simulink model "trajectory_traking"  (R2022b)
settings: Solver=ode4  StartTime=0.0  StopTime=T-T/duration  FixedStep=T/duration  RelTol=1e-3
values from neighbouring files (symbols this model uses):
  A = [ ... (first row only)    [path_generation.m]    (also in pid_test.m; trajectory.m)
  B = [ ... (first row only)    [path_generation.m]    (also in pid_test.m; trajectory.m)
  C = eye(4)    [path_generation.m]    (also in pid_test.m; trajectory.m)
  D = zeros(4,2)    [path_generation.m]    (also in pid_test.m; trajectory.m)
  Kd = 10*eye(4,2)    [drone.m]    (also in path_generation.m = K(:,3:4); trajectory.m = K(:,3:4))
  Kp = 20*eye(4,2)    [drone.m]    (also in path_generation.m = K(:,1:2); trajectory.m = K(:,1:2))
  x0 = [ ... (first row only)    [path_generation.m]    (also in trajectory.m = X(1))
  y0 = Y(1)    [trajectory.m]
settings Model: Creator=simonecarena  LastModifiedBy=simonecarena

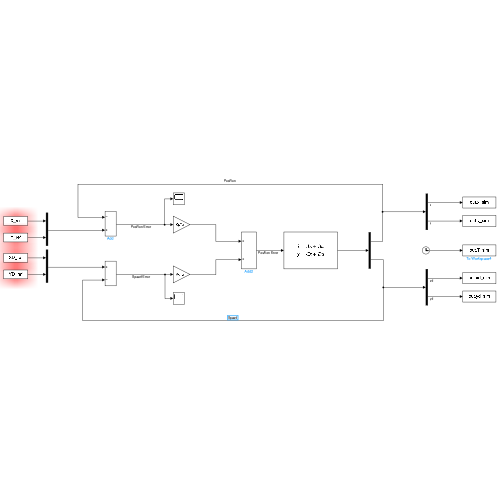
[thumbnail: Simulink's stored preview of the top-level diagram]
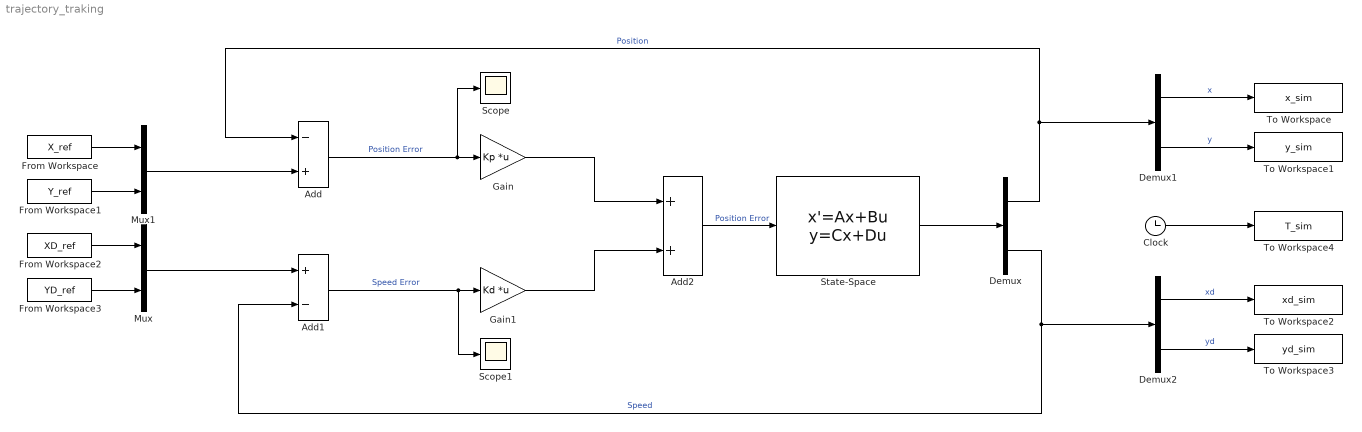
== system trajectory_traking ==
  Add : Sum  Inputs=-+
  Add1 : Sum  Inputs=+-
  Add2 : Sum
  Clock : Clock
  Demux : Demux  Outputs=2
  Demux1 : Demux  Outputs=2
  Demux2 : Demux  Outputs=2
  From Workspace : FromWorkspace  VariableName=X_ref  OutDataTypeStr=double
  From Workspace1 : FromWorkspace  VariableName=Y_ref  OutDataTypeStr=double
  From Workspace2 : FromWorkspace  VariableName=XD_ref  OutDataTypeStr=double
  From Workspace3 : FromWorkspace  VariableName=YD_ref  OutDataTypeStr=double
  Gain : Gain  Gain=Kp  Multiplication=Matrix(K*u)
  Gain1 : Gain  Gain=Kd  Multiplication=Matrix(K*u)
  Mux : Mux  Inputs=2
  Mux1 : Mux  Inputs=2
  Scope : Scope
  Scope1 : Scope
  State-Space : StateSpace  A=A  B=B  C=C  D=D  InitialCondition=[x0;y0;0;0]
  To Workspace : ToWorkspace  VariableName=x_sim  SampleTime=-1
  To Workspace1 : ToWorkspace  VariableName=y_sim  SampleTime=-1
  To Workspace2 : ToWorkspace  VariableName=xd_sim  SampleTime=-1
  To Workspace3 : ToWorkspace  VariableName=yd_sim  SampleTime=-1
  To Workspace4 : ToWorkspace  VariableName=T_sim  SampleTime=-1
  wires:
  Mux/1 -> Add1/1
  Mux1/1 -> Add/2
  State-Space/1 -> Demux/1
  Demux/1 -> Demux1/1, Add/1  "Position"
  Demux/2 -> Demux2/1, Add1/2  "Speed"
  Add/1 -> Scope/1, Gain/1  "Position Error"
  Add1/1 -> Scope1/1, Gain1/1  "Speed Error"
  Gain/1 -> Add2/1
  Gain1/1 -> Add2/2
  Add2/1 -> State-Space/1  "Position Error"
  Demux1/1 -> To Workspace/1  "x"
  Demux1/2 -> To Workspace1/1  "y"
  Demux2/2 -> To Workspace3/1  "yd"
  Demux2/1 -> To Workspace2/1  "xd"
  Clock/1 -> To Workspace4/1
  From Workspace2/1 -> Mux/1
  From Workspace3/1 -> Mux/2
  From Workspace/1 -> Mux1/1
  From Workspace1/1 -> Mux1/2
